simulink model "dianlu"  (Simulink 3.00)
settings: Solver=ode45  StartTime=0.0  StopTime=15.0  RelTol=1e-3
values from neighbouring files (symbols this model uses):
  C = [ 0    2 ... (first row only)    [csfunc.m]    (also in dsfunc.m = [      0    2.0761; initial.m = 0.32)
  L = 2    [initial.m]
  R = 1.4    [initial.m]
  Vs = 1    [initial.m]
libraries: simulink3 x1

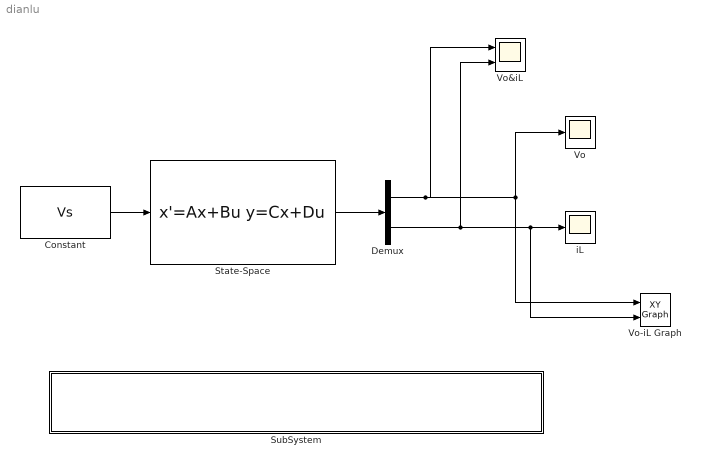
== system dianlu ==
  Constant : Constant  Value=Vs
  Demux : Demux  Outputs=2
  State-Space : StateSpace  A=[0 1/C;-1/L -R/L]  B=[0;1/L]  C=[1 0;0 1]  D=[0;0]  X0=[0.5;0]
  SubSystem : Subsystem
      settings: OpenFcn=initial
      mask Display: disp('Before Simulation,Double click here\nLoading initial Parameter:Vs,C,R,L')
  Vo : Scope
      settings: TimeRange=15  YMin=0.5  YMax=1.3  SaveToWorkspace=off  SaveName=ScopeData
  Vo&iL : Scope  NumInputPorts=2
      settings: TimeRange=15  YMin=-0.2~-5  YMax=1.2~5  SaveToWorkspace=off  SaveName=ScopeData
  Vo-iL Graph : simulink3/Sinks/XY Graph  xmin=0.4  xmax=1.3  ymin=-0.1  ymax=0.15  st=-1
  iL : Scope
      settings: TimeRange=15  YMin=-0.1  YMax=0.15  SaveToWorkspace=off  SaveName=ScopeData
  wires:
  Constant/1 -> State-Space/1
  State-Space/1 -> Demux/1
  Demux/1 -> Vo/1, Vo-iL Graph/1, Vo&iL/1
  Demux/2 -> iL/1, Vo-iL Graph/2, Vo&iL/2

== system dianlu/SubSystem ==
